simulink model "suivi_ligne_huit_2022_eleve_2022b"  (R2023b)
settings: Solver=VariableStepAuto  StartTime=0.0  StopTime=300  RelTol=1e-3
InitFcn:
  | close all;
libraries: mobileRoboticsLib x2, visionsources x2, dspvision x2, visionsinks x2
settings Model: Creator=Caroline Lelandais  LastModifiedBy=julienletzelter
settings SolverCC: AlgebraicLoopSolver=TrustRegion
settings OptimizationCC: ReuseModelBlockBuffer=off
settings DebuggingCC: UnconnectedInputMsg=warning  UnconnectedOutputMsg=warning  UnconnectedLineMsg=warning
settings ModelReferenceCC: EnableRefExpFcnMdlSchedulingChecks=on

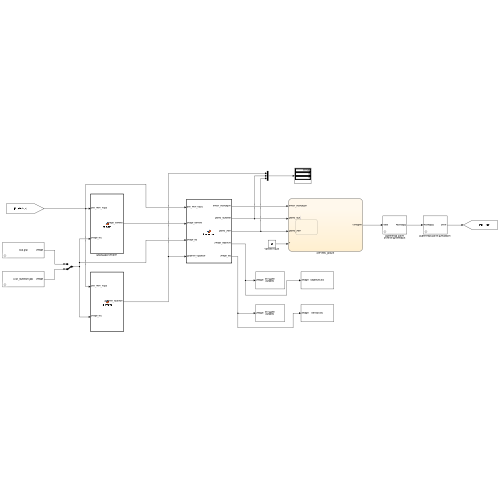
[thumbnail: Simulink's stored preview of the top-level diagram]
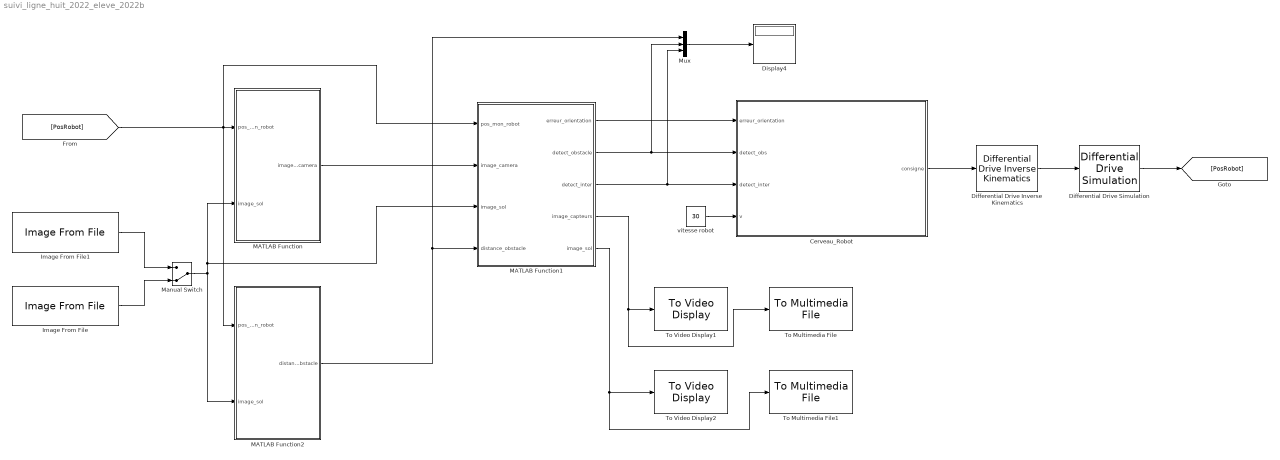
== system suivi_ligne_huit_2022_eleve_2022b ==
  Cerveau_Robot : Stateflow chart  TreatAsAtomicUnit=on
  Differential Drive Inverse Kinematics : mobileRoboticsLib/Kinematic Models/Differential Drive/Differential Drive Inverse Kinematics  wheelRadius=0.1  wheelBase=0.5
      settings: SourceProductName=Mobile Robotics Simulation Toolbox
  Differential Drive Simulation : mobileRoboticsLib/Kinematic Models/Differential Drive/Differential Drive Simulation  wheelRadius=0.1  wheelBase=0.5  initX=291  initY=451  initAngle=2.4  Ts=0.1
      settings: SourceProductName=Mobile Robotics Simulation Toolbox
  Display4 : Display
  Image From File : visionsources/Image From File  Tag=vipblks_nd  FileName=huit_obstacle.jpg  Ts=inf  imagePorts=One multidimensional signal  OutPortLabels=R|G|B  ImageDataType=Inherit from input image  sdImageDataType=uint(8)  Signed=on  WordLength=16  FractionLengthMode=User-defined  FractionLength=15
  Image From File1 : visionsources/Image From File  Tag=vipblks_nd  FileName=huit.jpg  Ts=inf  imagePorts=One multidimensional signal  OutPortLabels=R|G|B  ImageDataType=Inherit from input image  sdImageDataType=uint(8)  Signed=on  WordLength=16  FractionLengthMode=User-defined  FractionLength=15
  MATLAB Function : MATLAB Function  TreatAsAtomicUnit=on
  MATLAB Function1 : MATLAB Function  TreatAsAtomicUnit=on
  MATLAB Function2 : MATLAB Function  TreatAsAtomicUnit=on
  Manual Switch : ManualSwitch  CurrentSetting=0
  Mux : Mux  Inputs=3
  To Multimedia File : dspvision/To Multimedia File  outputFilename=capteurs.avi  streamSelection=Video only  videoCompressor=None (uncompressed)  audioCompressor=None (uncompressed)  imagePorts=One multidimensional signal  fileType=AVI  audioDatatype=Determine from input data type  fourcc=RGB  videoQuality=75  mj2000CompFactor=10
  To Multimedia File1 : dspvision/To Multimedia File  outputFilename=terrain.avi  streamSelection=Video only  videoCompressor=None (uncompressed)  audioCompressor=None (uncompressed)  imagePorts=One multidimensional signal  fileType=AVI  audioDatatype=Determine from input data type  fourcc=RGB  videoQuality=75  mj2000CompFactor=10
  To Video Display1 : visionsinks/To Video Display  windowSizeMode=Normal  openAtMdlStart=on  fullScreen=off  videoWindowX=536805376  videoWindowY=536805376  saveWindowSize=off  videoWindowWidth=520  videoWindowHeight=352  inputColorFormat=RGB  inputType=Obsolete  imagePorts=One multidimensional signal  OutputDevice=On-screen video monitor  dataOrg=Column-major  isWindowOpen=off
  To Video Display2 : visionsinks/To Video Display  windowSizeMode=Normal  openAtMdlStart=on  fullScreen=off  videoWindowX=16  videoWindowY=88  saveWindowSize=off  videoWindowWidth=1247  videoWindowHeight=642  inputColorFormat=RGB  inputType=Obsolete  imagePorts=One multidimensional signal  OutputDevice=On-screen video monitor  dataOrg=Column-major  isWindowOpen=off
  vitesse robot : Constant  Value=30
  wires:
  Differential Drive Inverse Kinematics/1 -> Differential Drive Simulation/1
  Cerveau_Robot/1(consigne) -> Differential Drive Inverse Kinematics/1
  Differential Drive Simulation/1 -> [PosRobot]
  [PosRobot] -> MATLAB Function1/1(pos_mon_robot), MATLAB Function2/1(pos_mon_robot), MATLAB Function/1(pos_mon_robot)
  vitesse robot/1 -> Cerveau_Robot/4(v)
  MATLAB Function1/1(erreur_orientation) -> Cerveau_Robot/1(erreur_orientation)
  MATLAB Function1/2(detect_obstacle) -> Mux/2, Cerveau_Robot/2(detect_obs)
  MATLAB Function1/3(detect_inter) -> Mux/3, Cerveau_Robot/3(detect_inter)
  MATLAB Function1/4(image_capteurs) -> To Video Display1/1, To Multimedia File/1
  MATLAB Function1/5(image_sol) -> To Video Display2/1, To Multimedia File1/1
  MATLAB Function2/1(distance_obstacle) -> Mux/1, MATLAB Function1/4(distance_obstacle)
  MATLAB Function/1(image_camera) -> MATLAB Function1/2(image_camera)
  Manual Switch/1 -> MATLAB Function1/3("image_sol "), MATLAB Function/2(image_sol), MATLAB Function2/2(image_sol)
  Image From File1/1 -> Manual Switch/1
  Image From File/1 -> Manual Switch/2
  Mux/1 -> Display4/1

== matlab function suivi_ligne_huit_2022_eleve_2022b/MATLAB Function ==
  data: pos_mon_robot input; image_sol input; image_camera output
% Son rôle est de modéliser la photo brute prise par la caméra. Le modèle est extrêmement simplifié et fait comme si la photo était prise à la verticale et à l’avant du robot (par d’angle de vue).
% •	Entrées : pos_mon_robot (position du robot), image_sol (« terrain » soit la vue du ciel du circuit où doit évoluer le robot )
% •	Sorties : image_camera (vue du ciel du champ de vision du robot, rectangle rouge sur Video Display2)



function image_camera  = camera(pos_mon_robot, image_sol)

% Caractéristiques des coordonnées du champ de vision de la caméra 
profondeur_camera = 40;
demi_largeur_camera = 15;

% Récupération de la position du robot concerné
pos_x_vehicule = round(pos_mon_robot(1));
pos_y_vehicule = round(pos_mon_robot(2));
pos_angle_vehicule = pos_mon_robot(3);

%image vue par le capteur
image_camera=uint8(zeros(profondeur_camera,2*demi_largeur_camera,3));
for i=1:profondeur_camera
    for j=1:2*demi_largeur_camera
        c=(pos_x_vehicule+1j*pos_y_vehicule)+(i+1j*(j-demi_largeur_camera))*exp(1j*pos_angle_vehicule);
        image_camera(i,j,:)=image_sol(round(real(c)),round(imag(c)),:);
    end
end

== matlab function suivi_ligne_huit_2022_eleve_2022b/MATLAB Function2 ==
  data: pos_mon_robot input; image_sol input; distance_obstacle output
% Son rôle est de modéliser le signal de sortie du télémètre à l’avant du robot.
% •	Entrées : pos_mon_robot (position du robot), image_sol (« terrain » soit la vue du ciel du circuit où doit évoluer le robot )
% •	Sorties : distance_obstacle (distance de l’obstacle)


function distance_obstacle    = telemetre(pos_mon_robot, image_sol)

% Caractéristiques des coordonnées du champ de vision du télémètre

profondeur_telemetre_x = 80;
largeur_telemetre_y = 5;

% Récupération de la position du robot concerné
pos_x_vehicule = round(pos_mon_robot(1));
pos_y_vehicule = round(pos_mon_robot(2));
pos_angle_vehicule = pos_mon_robot(3);

%image vue par le capteur et detection d'un obstacle
image_capteur2=uint8(zeros(profondeur_telemetre_x,2*largeur_telemetre_y,3));
distance_obstacle=100000;
for i=1:profondeur_telemetre_x
    for j=1:2*largeur_telemetre_y
        c=(pos_x_vehicule+1j*pos_y_vehicule)+(i+1j*(j-largeur_telemetre_y))*exp(1j*pos_angle_vehicule);
        image_capteur2(i,j,:)=image_sol(round(real(c)),round(imag(c)),:);
        if (image_capteur2(i,j,1)>200) && (image_capteur2(i,j,2)<50) && (image_capteur2(i,j,3)<50)   % obstacle simulé ici par couleur rouge
            distance_obstacle=min(distance_obstacle,abs((i+1j*j)-(0+1j*largeur_telemetre_y)));
        end
    end
end

== stateflow chart suivi_ligne_huit_2022_eleve_2022b/Cerveau_Robot ==
  state SuivreLigne
    angle_dir=erreur_orientation;
    w = angle_dir;%algo reliant l'erreur d'orientation du robot à la consigne de vitesse angulaire
    consigne = [v;w];
  state Arret
    consigne = [0;90];
  (default) -> SuivreLigne
  Arret -> SuivreLigne : [detect_obs ==0]
  SuivreLigne -> Arret : [detect_obs ==1]
  data: consigne output; w local; angle_dir local; erreur_orientation input; detect_obs input; detect_inter input; v input

== matlab function suivi_ligne_huit_2022_eleve_2022b/MATLAB Function1 ==
  data: pos_mon_robot input; image_camera input; erreur_orientation output; detect_obstacle output; detect_inter output; image_sol input; image_capteurs output; image_sol output; distance_obstacle input
% Ce bloc doit analyser les données venant des capteurs pour en extraire les informations d’erreur d’orientation du robot, détection d’un obstacle et détection d’une intersection. 
% Ce bloc permet aussi la génération d’une animation video montrant l’évolution du robot sur le terrain et la vision du robot (figure 1).
% •	Entrées : pos_mon_robot, image_camera, distance_obstacle, image_sol
% •	Sorties : erreur_orientation (scalaire modélisant l’erreur signée de l’axe du robot par rapport à celui de la ligne), detect_obstacle (à 1 si obstacle) , detect_inter (à 1 si un croisement est détecté), image_capeurs, image_sol



function [erreur_orientation, detect_obstacle,detect_inter, image_capteurs,image_sol]  = Perception(pos_mon_robot,image_camera, image_sol,distance_obstacle)

% Caractéristiques des coordonnées du champ de vision de la caméra et du télémètre
profondeur_camera = 40;
demi_largeur_camera = 15;
profondeur_telemetre = 80;
demi_largeur_telemetre = 5;
longueur_robot=30;
demi_largeur_robot=10;

% Récupération de la position du robot concerné
pos_x_vehicule = round(pos_mon_robot(1));
pos_y_vehicule = round(pos_mon_robot(2));
pos_angle_vehicule = pos_mon_robot(3);

%Calcul de detect_obstacle : 

if distance_obstacle <= 2*longueur_robot
    detect_obstacle = 1;
else
    detect_obstacle = 0;
end

image_camera = image_camera(1:profondeur_camera,:,:);

function y = process(x)
    gray_image = rgb2gray(x);
    edges = edge(gray_image);
    y = edges;
end

im_closed = process(image_camera);

%%%%%%%%% HOUGH TRANSFORM %%%%%%%%%%%%%
    function [correct_angle,lines] = houghing(x,ref,n_lines,min_dist)
        [H,T,R] = hough( x, 'Theta', -90:1:89, 'RhoResolution', 2.00 ); % pas = 2 pix;
        
        maxNumPeaks = n_lines;    % Maximum number of peaks
        threshold = 0.7;       % Minimum value to be considered a peak
        nHoodSize = [3 21];              % The neighborhood around each peak that is set to zero after the peak is identified
        
        P = houghpeaks( H, maxNumPeaks, 'threshold', threshold, 'NHoodSize', nHoodSize );       
        if not(isempty(P))
            mergeDistance = round(0.9*profondeur_camera);   % Line segments will be merged if distance between them is less than this
            minLength = round(min_dist*profondeur_camera);       % Minimum line length
            lines = houghlines( x, T, R, P, 'FillGap', mergeDistance, 'MinLength', minLength );
            
            for ii = 1:length(lines)                                            
	            xy = [lines(ii).point1; lines(ii).point2];
            end          
              if not(isempty(lines))
                  distance = lines(1,1).point2(1);
                  display(lines(1,1))
                  theta = lines(1,1).theta;
                  display(theta);
                  if theta > 0
                      sign = 1;
                  elseif theta < 0
                      sign = -1;
                  else
                      sign = 0;
                  end

                  if abs(distance - demi_largeur_camera) > demi_largeur_robot/2 && abs(theta) > 3
                      correct_angle = round(-(lines(1,1).theta)/6) + sign;
                  elseif abs(distance - demi_largeur_camera) > demi_largeur_robot/3
                      correct_angle = (distance - demi_largeur_camera)/abs(distance - demi_largeur_camera);
                  else
                      correct_angle = 0;
                  end
              else
                  correct_angle = 0;
              end
        else
            correct_angle = 0;
            lines = [];
        end
    end


n_lines = 4;
[erreur_orientation,test] = houghing(im_closed,demi_largeur_camera,n_lines,0.75);


[error,lines] = houghing(im_closed,0,6,0.2);
is_inter = 0;
angle_value=0;
l1 = 0;
l2 = 0;
if not(isempty(lines))
for kk=1:(size(lines,2)-1)
   for ll=kk+1:(size(lines,2))
       l1 = cat(2,[lines(kk).point1],[lines(kk).point2]);
       l2 = cat(2,[lines(ll).point1],[lines(ll).point2]);
       x1 = l1(1);
       y1 = l1(2);
       x2 = l1(3);
       y2 = l1(4);
       x3 = l2(1);
       y3 = l2(2);
       x4 = l2(3);
       y4 = l2(4);
       u = [x2,y2,0] - [x1,y1,0];
       v = [x4,y4,0] - [x3,y3,0];
       CosTheta = max(min(dot(u,v)/(norm(u)*norm(v)),1),-1);
        angle_value = real(acosd(CosTheta));
       %angle_value = angle_value * 180/pi;
%        angle_value = abs(mod((atan((l2(4)-l2(2))/(l2(3)-l2(1)))- atan((l1(4)-l1(2))/(l1(3)-l1(1))) * 180/pi),180)-90);
       if angle_value >= 80
           is_inter = 1;
       end
   end
end
else
is_inter = 0;
end
%[error,lines] = houghing(im_closed,0,6,0.2);

%%%%%%%%%%%%%%%%%%%%%%%%%%%%%  différentes erreurs à estimer  %%%%%%%%%%%%%%%%%%%%%%%%%%%%%%%%%%%%%%%%%%%%
%erreur_orientation=0; % à déterminer avec l'image envoyée par la caméra
detect_inter=0;  %=1 si détection d'une intersection
%%%%%%%%%%%%%%%%%%%%%%%%%%%%%%%%%%%%%%%%%%%%%%%%%%%%%%%%%%%%%%%%%%%%%%%%%%%%%%%%%%%%%%%%%%%%%%%%%%%%%%%%%%




%dessin de la sone de vision = de ce que voient les 2 capteurs
image_capteurs=uint8(zeros(80,30,3));
image_capteurs(1:profondeur_camera,1:2*demi_largeur_camera,:)=image_camera;
for i=profondeur_camera+1:profondeur_telemetre
   for j=1:2*demi_largeur_camera
       c=(pos_x_vehicule+1j*pos_y_vehicule)+(i+1j*(j-demi_largeur_camera))*exp(1j*pos_angle_vehicule);
       image_capteurs(i,j,:)=image_sol(round(real(c)),round(imag(c)),:);
   end
end



%dessin sur le terrain du robot en vert
for i=1:longueur_robot
    for j=1:2*demi_largeur_robot
        c=(pos_x_vehicule+1j*pos_y_vehicule)-(i+1j*(j-demi_largeur_robot))*exp(1j*pos_angle_vehicule);
        image_sol(round(real(c)),round(imag(c)),2)=255;
    end
end

%dessin sur le terrain de la zone de vision de la caméra en rouge
for i=1:profondeur_camera
    for j=1:2*demi_largeur_camera
        c=(pos_x_vehicule+1j*pos_y_vehicule)+(i+1j*(j-demi_largeur_camera))*exp(1j*pos_angle_vehicule);
        image_sol(round(real(c)),round(imag(c)),1)=255;
    end
end

%dessin sur le terrain de la zone de vision du télémètre en bleu
for i=1:profondeur_telemetre
    for j=1:2*demi_largeur_telemetre
        c=(pos_x_vehicule+1j*pos_y_vehicule)+(i+1j*(j-demi_largeur_telemetre))*exp(1j*pos_angle_vehicule);
        image_sol(round(real(c)),round(imag(c)),3)=255;
    end
end

%dessin (sur le terrain et sur la zone de vision) du point estimé par traitement image ; si la détection de ligne se passe bien le point doit rester sur la ligne 
%ici ce point est représenté à mi-profondeur de la vision de la caméra mais cela peut être modifié suiva t l'lagorithme utilisé
point_estime=(pos_x_vehicule+1j*pos_y_vehicule)+(profondeur_camera/2+1j*(erreur_orientation))*exp(1j*pos_angle_vehicule);
NoLigne=round(real(point_estime));NoColonne=round(imag(point_estime));
image_sol(NoLigne-2:NoLigne+2,NoColonne-2:NoColonne+2,2)=255;  
if abs(erreur_orientation)<demi_largeur_camera-2
    image_capteurs(round(profondeur_camera/2)-2:round(profondeur_camera/2)+2,demi_largeur_camera+erreur_orientation-2:demi_largeur_camera+erreur_orientation+2,2)=255;
end




%tracé des contours 
% des capteurs  (caméra en rouge ; télémètre en bleu)
image_capteurs(1,:,1)=240;   %bas
image_capteurs(1:profondeur_camera,1,1)=240;   %droite
image_capteurs(profondeur_camera,:,1)=240; %haut
image_capteurs(1:profondeur_camera,end,1)=240; %gauche
image_capteurs(1,demi_largeur_camera-demi_largeur_telemetre:end-(demi_largeur_camera-demi_largeur_telemetre),3)=240;   %bas
image_capteurs(:,demi_largeur_camera-demi_largeur_telemetre,3)=240;   %droite
image_capteurs(end,demi_largeur_camera-demi_largeur_telemetre:end-(demi_largeur_camera-demi_largeur_telemetre),3)=240; %haut
image_capteurs(:,end-(demi_largeur_camera-demi_largeur_telemetre),3)=240; %gauche
image_capteurs=flipud(image_capteurs);
image_capteurs=fliplr(image_capteurs);

%du terrain
image_sol(1:2,:,3)=240; 
image_sol(:,1:2,3)=240;
image_sol(end-1:end,:,3)=240;
image_sol(:,end-1:end,3)=240;
image_sol(pos_x_vehicule-1:pos_x_vehicule+1,pos_y_vehicule-1:pos_y_vehicule+1,2)=255;

end
